simulink model "Setpoint_Open"  (R2024a)
settings: Solver=FixedStepAuto  StartTime=0.0  StopTime=Inf  FixedStep=Ts  RelTol=RelativeTolerance  EnableMultiTasking=on
libraries: c2802xlib x1, c2837xDlib x1
settings Model: ExtModeTrigDuration=8  Creator=Fernand  LastModifiedBy=cesar
settings DataIOCC: SaveFormat=StructureWithTime  ReturnWorkspaceOutputs=off  OutputSaveName=data_results  SignalLoggingName=DataResult
settings OptimizationCC: DefaultUnderspecifiedDataType=single  EnhancedBackFolding=on  PassReuseOutputArgsAs=Individual arguments  MaxStackSize=1024  OptimizeBlockOrder=speed  DifferentSizesBufferReuse=on  OptimizationCustomize=off  EfficientTunableParamExpr=on
settings DebuggingCC: ParameterTunabilityLossMsg=error
settings HardwareCC: ProdBitPerChar=16  ProdBitPerInt=16  ProdBitPerPointer=32  ProdBitPerSizeT=32  ProdBitPerPtrDiffT=32  ProdLargestAtomicInteger=Integer  ProdLargestAtomicFloat=None  ProdWordSize=16  ProdLongLongMode=on  ProdHWDeviceType=Texas Instruments->C2000  HardwareBoardFeatureSet=SoCBlockset
settings ModelReferenceCC: ModelReferenceNumInstancesAllowed=Single
settings SFSimCC: MATLABDynamicMemAlloc=off
settings RTWCC: Description=Embedded Coder  SystemTargetFile=ert.tlc  HardwareBoard=TI Delfino F28379D LaunchPad  TemplateMakefile=ert_default_tmf  Toolchain=Texas Instruments Code Composer Studio (C2000)  CodeProfilingSaveOptions=MetricsOnly  GPUComputeCapability=3.5
settings CodeAppCC: ForceParamTrailComments=on  IgnoreCustomStorageClasses=off  OperatorAnnotations=on  SimulinkDataObjDesc=on  SFDataObjDesc=on  InsertBlockDesc=on
settings ERTTargetCC: CodeReplacementLibrary=TI C28x  ExtModeTransport=4  ExtModeStaticAlloc=on  ExtModeAutomaticAllocSize=off  ExtModeStaticAllocSize=10000  ExtModeMexFile=ext_xcp  ExtModeIntrfLevel=Level2 - Open

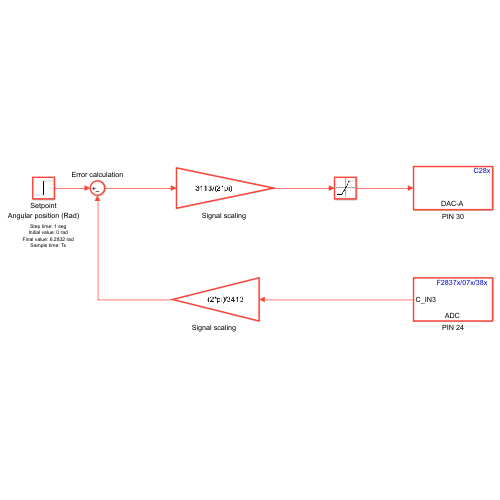
[thumbnail: Simulink's stored preview of the top-level diagram]
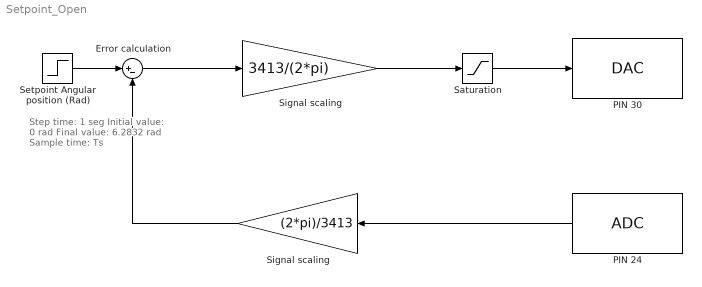
== system Setpoint_Open ==
  note: Step time: 1 seg
      | Initial value: 0 rad
      | Final value: 6.2832 rad
      | Sample time: Ts
  Error calculation : Sum  Inputs=|+-
  PIN 24 : c2802xlib/ADC  blkParamProc=C2000_Type4  ADCModule=C  samplingMode=Single sample mode  ADCResolution=12-bit (Single-ended input)  useSOC1=SOC0  useSOC2=SOC0_SOC1  SOCAcquisitionWindow=15  SOCTriggerSource=Software  SOCInterruptTrigger=No ADCINT  Ts=-1  dType=uint16  postInterrupt=off  interruptSel=ADCINT1  ADCINTContinuous=on  endma=off  chdma=1  conv1=ADCINA0  conv2=ADCINA0 and ADCINB0  conv1_Type4=ADCIN3  conv2_Type4=ADCIN0 and ADCIN1
      settings: LibrarySourceBlock=c2837xDlib/ADC
  PIN 30 : c2837xDlib/DAC  channel=A  saturate=off
  Saturation : Saturate  UpperLimit=3413  LowerLimit=0
  Setpoint Angular position (Rad) : Step  After=2*pi
  "Signal scaling " : Gain  Gain=3413/(2*pi)
  "Signal scaling  " : Gain  Gain=(2*pi)/3413  OutDataTypeStr=double
  wires:
  Setpoint Angular position (Rad)/1 -> Error calculation/1
  "Signal scaling  "/1 -> Error calculation/2
  "Signal scaling "/1 -> Saturation/1
  Error calculation/1 -> "Signal scaling "/1
  PIN 24/1 -> "Signal scaling  "/1
  Saturation/1 -> PIN 30/1
